simulink model "Simulink2017"  (R2017a)
settings: Solver=VariableStepAuto  StartTime=0.0  StopTime=20.0  RelTol=1e-3
values from neighbouring files (symbols this model uses):
  A = [0 1 1 1 1 1 ... (first row only)    [Initial.m]    (also in matlab_promjena_form.mat = [0 1 1 1 1 1 0 1 1 1 1 1 ... (25 elements, 5x5)])
  B = [0 1 1 1 1 1 ... (first row only)    [Initial.m]
  C = [0 1 1 1 1 1 ... (first row only)    [Initial.m]
  R = [10, 5, -5, -10, -5 , 5 ; 0, 5*sqrt(3), 5*sqrt(3), 0, -5*sqrt(3),-5*sqrt(3) ]    [Initial.m]
  vxd = -1    [Initial.m]
  vyd = -1    [Initial.m]
  x0 = [0, 30, 10, 60, 20, 0]    [Initial.m]    (also in matlab_promjena_form.mat = [0 -1 -1 -2 -2])
  y0 = [30, 60, 50, 40, 100, 100]    [Initial.m]    (also in matlab_promjena_form.mat = [0 1 -1 2 -2])
settings Model: Creator=Mare  LastModifiedBy=Mare

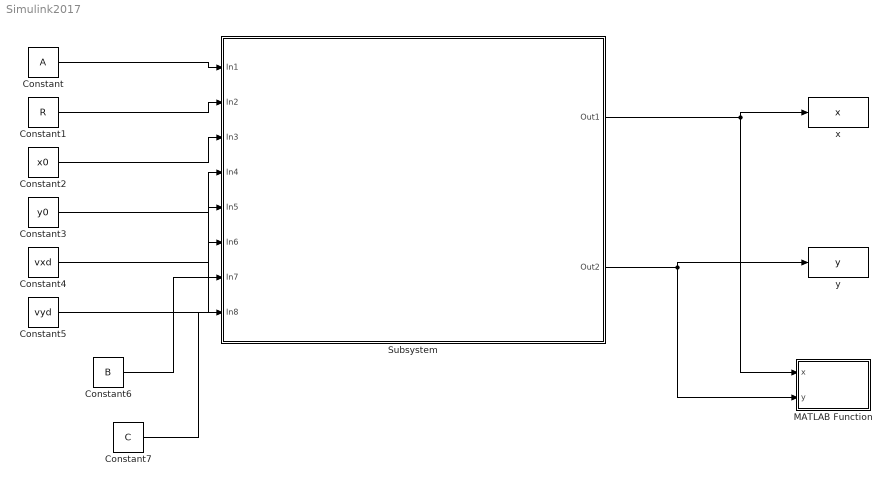
== system Simulink2017 ==
  Constant : Constant  Value=A
  Constant1 : Constant  Value=R
  Constant2 : Constant  Value=x0
  Constant3 : Constant  Value=y0
  Constant4 : Constant  Value=vxd
  Constant5 : Constant  Value=vyd
  Constant6 : Constant  Value=B
  Constant7 : Constant  Value=C
  MATLAB Function : MATLAB Function  TreatAsAtomicUnit=on
  Subsystem : Subsystem
  x : ToWorkspace  VariableName=x  SaveFormat=Structure With Time  SampleTime=0.5
  y : ToWorkspace  VariableName=y  SaveFormat=Structure With Time  SampleTime=0.5
  wires:
  Subsystem/1(Out1) -> x/1, MATLAB Function/1(x)
  Subsystem/2(Out2) -> y/1, MATLAB Function/2(y)
  Constant3/1 -> Subsystem/4(In4)
  Constant2/1 -> Subsystem/3(In3)
  Constant1/1 -> Subsystem/2(In2)
  Constant/1 -> Subsystem/1(In1)
  Constant4/1 -> Subsystem/5(In5)
  Constant5/1 -> Subsystem/6(In6)
  Constant6/1 -> Subsystem/7(In7)
  Constant7/1 -> Subsystem/8(In8)

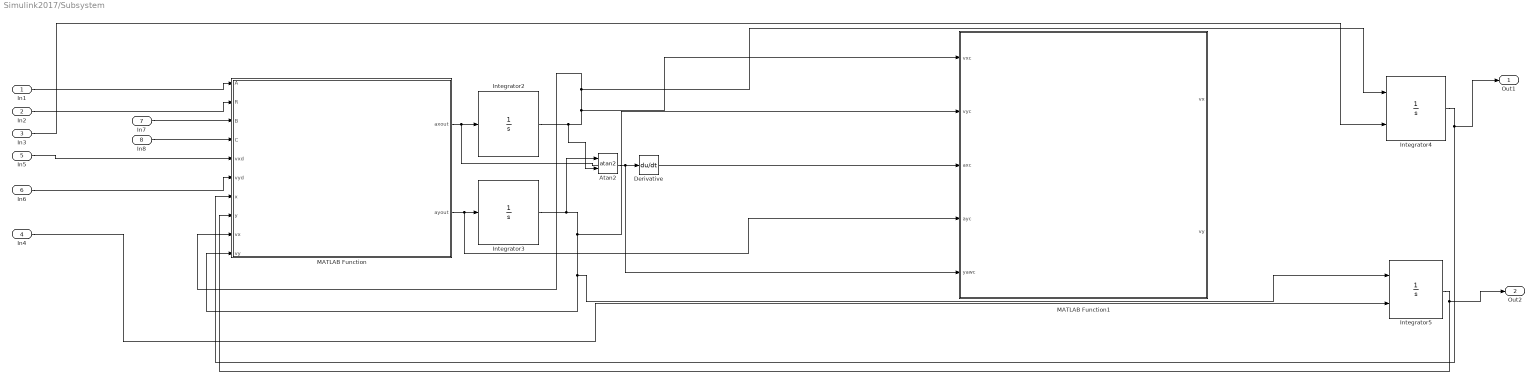
== system Simulink2017/Subsystem ==
  In1 : Inport
  In2 : Inport  Port=2
  In3 : Inport  Port=3
  In4 : Inport  Port=4
  In5 : Inport  Port=5
  In6 : Inport  Port=6
  In7 : Inport  Port=7
  In8 : Inport  Port=8
  Atan2 : Trigonometry  Operator=atan2
  Derivative : Derivative
  Integrator2 : Integrator
  Integrator3 : Integrator
  Integrator4 : Integrator  InitialConditionSource=external
  Integrator5 : Integrator  InitialConditionSource=external
  MATLAB Function : MATLAB Function  TreatAsAtomicUnit=on
  MATLAB Function1 : MATLAB Function  TreatAsAtomicUnit=on
  Out1 : Outport
  Out2 : Outport  Port=2
  wires:
  In1/1 -> MATLAB Function/1(A)
  In2/1 -> MATLAB Function/2(R)
  In3/1 -> Integrator4/2
  In4/1 -> Integrator5/2
  MATLAB Function/1(axout) -> MATLAB Function1/3(axc), Integrator2/1
  MATLAB Function/2(ayout) -> MATLAB Function1/4(ayc), Integrator3/1
  Integrator3/1 -> Atan2/1, MATLAB Function1/2(vyc), Integrator5/1, MATLAB Function/10(vy)
  Integrator2/1 -> Atan2/2, MATLAB Function1/1(vxc), Integrator4/1, MATLAB Function/9(vx)
  In5/1 -> MATLAB Function/5(vxd)
  In6/1 -> MATLAB Function/6(vyd)
  In8/1 -> MATLAB Function/4(C)
  In7/1 -> MATLAB Function/3(B)
  Atan2/1 -> MATLAB Function1/5(yawc), Derivative/1
  Integrator4/1 -> Out1/1, MATLAB Function/7(x)
  Integrator5/1 -> Out2/1, MATLAB Function/8(y)

== matlab function Simulink2017/Subsystem/MATLAB Function ==
  data: axout output; A input; ayout output; R input; B input; C input; vxd input; vyd input; x input; y input; vx input; vy input
function [axout, ayout]  = fcn(A, R, B, C, vxd, vyd ,x,y,vx,vy)
axout=zeros(length(A),1);
ayout = zeros(length(A),1);
%azout = zeros(length(A),1);

for i = 1:length(A)
    axout(i) = 0 - (vx(i)-vxd);
    ayout(i) = 0 - (vy(i)-vyd);
    %azout(i) = 0 - C(i)*vz(i);
    for j = 1:length(A)
        axout(i) = axout(i) - A(i,j)*((x(i)-R(1,i))-(x(j)-R(1,j))+ (vx(i)-vx(j)));
        ayout(i) = ayout(i) - A(i,j)*((y(i)-R(2,i))-(y(j)-R(2,j))+ (vy(i)-vy(j)));
        %azout(i) = azout(i) - A(i,j)*(B(j)*(z(i)-R(3,i))-(y(j)-R(3,j))+ C(j)*(vz(i)-vz(j)));
    end
end

== matlab function Simulink2017/MATLAB Function ==
  data: x input; y input
function  fcn(x,y)
%postavljanje granicnih vrijednosti koordinata
xmax = 300;
xmin = -100;
ymax = 300;
ymin = -100;

colors = {[0.6,0.9,0.6],[0,0.7,1],[0.85, 0.6,0.85],[1,0.8,0],[0.9,0.6,0.5], [0,1,0],[1,0,0]};


cla;
axis([xmin,xmax,ymin,ymax]);
xlabel('x');
ylabel('y');
grid on;

for k = 1:length(x)
    plot(x(k),y(k),'o', 'Color', colors{k});
    hold on;
end

coder.extrinsic('legend');
legend('a1', 'a2', 'a3', 'a4','a5','a6');

== matlab function Simulink2017/Subsystem/MATLAB Function1 ==
  data: vxc input; vx output; vyc input; axc input; ayc input; yawc input; vy output
function [vx,vy] = fcn(vxc,vyc,axc,ayc,yawc)
vx= zeros(1, 6);
vy = zeros(1, 6);
vi = sqrt(vxc.^2+vyc.^2)-sqrt(axc.^2+ayc.^2);

for i = 1:length(vxc)
    vx(i) = vi(i)*cos(yawc(i));
    vy(i) = vi(i)*sin(yawc(i));
end
